simulink model "PID_RS"  (R2019a)
settings: Solver=VariableStepAuto  StartTime=0.0  StopTime=10.0  RelTol=1e-3
values from neighbouring files (symbols this model uses):
  f = 7E-5    (= 7e-05)    [BallOnBeam.m]
  J = 4.6E-5    (= 4.6e-05)    [BallOnBeam.m]
  k = 0.026    [BallOnBeam.m]
  k1 = 7    [BallOnBeam.m]
  k2 = 28.65    [BallOnBeam.m]
  k3 = 0.0159    [BallOnBeam.m]
  kb = 6.1    [BallOnBeam.m]
  ki = 1.6    [BallOnBeam.m]
  kp = nm*J*wndes^2/(k2*k*ki)    (= 27.0462934428)    [BallOnBeam.m]
  kpi = rm*tii*ki/taudesi    (= 1.6)    [BallOnBeam.m]
  kv = (2*xides*J*wndes - f)/(kp*ki*k*k3)    (= 0.093347474441)    [BallOnBeam.m]
  lm = 0.001    [BallOnBeam.m]
  nm = 960    [BallOnBeam.m]
  r0 = x(3)    [BallOnBeam.m]
  r1 = x(4)    [BallOnBeam.m]
  r2 = x(5)    [BallOnBeam.m]
  rm = 0.33    [BallOnBeam.m]
  s1 = x(2)    [BallOnBeam.m]
  Te = 0.2    [BallOnBeam.m]
  tii = 0.5*lm/rm    (= 0.00151515151515)    [BallOnBeam.m]
settings Model: Creator=DELL  LastModifiedBy=DELL

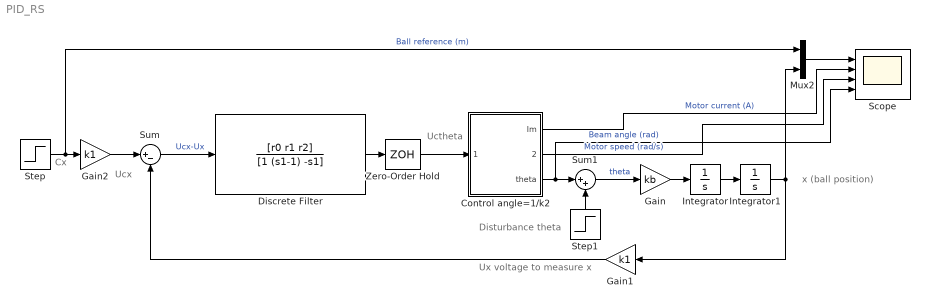
== system PID_RS ==
  note: x (ball position)
  note: Cx
  note: Ucx
  note: Uctheta
  note: Disturbance theta
  note: Ux voltage to measure x
  "Control angle=1/k2 " : Subsystem
  Discrete Filter : DiscreteFilter  Numerator=[r0 r1 r2]  Denominator=[1 (s1-1) -s1]  SampleTime=Te
  Gain : Gain  Gain=kb
  Gain1 : Gain  Gain=k1  SaturateOnIntegerOverflow=on  OutDataTypeStr=Inherit: Same as input  ParamDataTypeStr=Inherit: Same as input
  Gain2 : Gain  Gain=k1  SaturateOnIntegerOverflow=on  OutDataTypeStr=Inherit: Same as input  ParamDataTypeStr=Inherit: Same as input
  Integrator : Integrator
  Integrator1 : Integrator
  Mux2 : Mux  Inputs=2
  Scope : Scope  NumInputPorts=4
  Step : Step  After=0.1  SampleTime=0
  Step1 : Step  Time=10  After=1*pi/180  SampleTime=0
  Sum : Sum  Inputs=|+-  SaturateOnIntegerOverflow=on  InputSameDT=on  OutDataTypeStr=Inherit: Same as first input
  Sum1 : Sum  Inputs=|++  SaturateOnIntegerOverflow=on  InputSameDT=on  OutDataTypeStr=Inherit: Same as first input
  Zero-Order Hold : ZeroOrderHold  SampleTime=-1
  wires:
  "Control angle=1/k2 "/3(theta) -> Scope/4, Sum1/1  "Beam angle (rad)"
  Gain2/1 -> Sum/1
  Step/1 -> Mux2/1, Gain2/1  "Ball reference (m)"
  Step1/1 -> Sum1/2
  Mux2/1 -> Scope/1
  "Control angle=1/k2 "/2(omega) -> Scope/3  "Motor speed (rad/s)"
  "Control angle=1/k2 "/1(Im) -> Scope/2  "Motor current (A)"
  Gain1/1 -> Sum/2
  Discrete Filter/1 -> Zero-Order Hold/1
  Zero-Order Hold/1 -> "Control angle=1/k2 "/1(Uctheta)
  Sum/1 -> Discrete Filter/1  "Ucx-Ux"
  Sum1/1 -> Gain/1  "theta"
  Gain/1 -> Integrator/1
  Integrator1/1 -> Gain1/1, Mux2/2
  Integrator/1 -> Integrator1/1

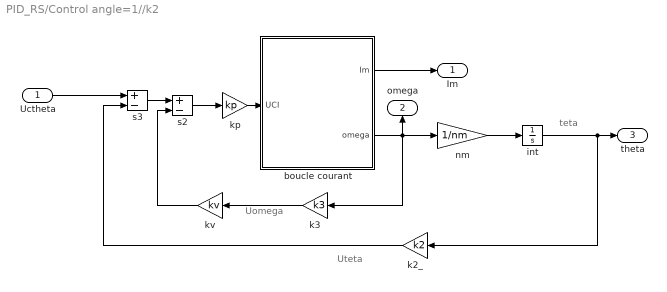
== system PID_RS/Control angle=1//k2  ==
  note: Uomega
  note: teta
  note: Uteta
  Uctheta : Inport
  boucle courant : Subsystem
  int : Integrator
  k2_ : Gain  Gain=k2  SaturateOnIntegerOverflow=on  OutDataTypeStr=Inherit: Same as input  ParamDataTypeStr=Inherit: Same as input
  k3 : Gain  Gain=k3  SaturateOnIntegerOverflow=on  OutDataTypeStr=Inherit: Same as input  ParamDataTypeStr=Inherit: Same as input
  kp : Gain  Gain=kp  SaturateOnIntegerOverflow=on  OutDataTypeStr=Inherit: Same as input  ParamDataTypeStr=Inherit: Same as input
  kv : Gain  Gain=kv  SaturateOnIntegerOverflow=on  OutDataTypeStr=Inherit: Same as input  ParamDataTypeStr=Inherit: Same as input
  nm : Gain  Gain=1/nm  SaturateOnIntegerOverflow=on  OutDataTypeStr=Inherit: Same as input  ParamDataTypeStr=Inherit: Same as input
  s2 : Sum  Inputs=+-  SaturateOnIntegerOverflow=on  InputSameDT=on  OutDataTypeStr=Inherit: Same as first input
  s3 : Sum  Inputs=+-  SaturateOnIntegerOverflow=on  InputSameDT=on  OutDataTypeStr=Inherit: Same as first input
  Im : Outport
  omega : Outport  Port=2
  theta : Outport  Port=3
  wires:
  kp/1 -> boucle courant/1(UCI)
  s2/1 -> kp/1
  s3/1 -> s2/1
  nm/1 -> int/1
  boucle courant/2(omega) -> nm/1, k3/1, omega/1
  k3/1 -> kv/1
  kv/1 -> s2/2
  int/1 -> k2_/1, theta/1
  k2_/1 -> s3/2
  boucle courant/1(Im) -> Im/1
  Uctheta/1 -> s3/1

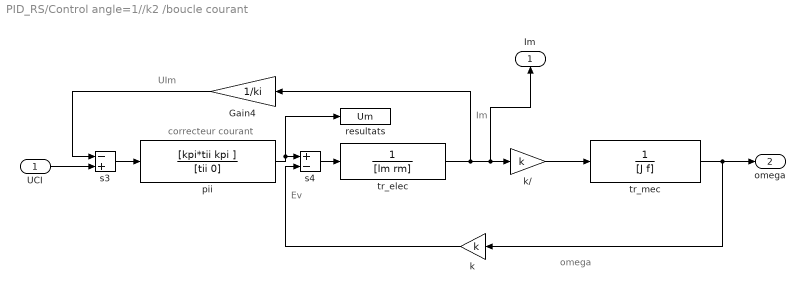
== system PID_RS/Control angle=1//k2 /boucle courant ==
  note: correcteur courant
  note: Im
  note: Ev
  note: UIm
  note: omega
  UCI : Inport
  Gain4 : Gain  Gain=1/ki  SaturateOnIntegerOverflow=on  OutDataTypeStr=Inherit: Same as input  ParamDataTypeStr=Inherit: Same as input
  k : Gain  Gain=k  SaturateOnIntegerOverflow=on  OutDataTypeStr=Inherit: Same as input  ParamDataTypeStr=Inherit: Same as input
  "k/ " : Gain  Gain=k  SaturateOnIntegerOverflow=on  OutDataTypeStr=Inherit: Same as input  ParamDataTypeStr=Inherit: Same as input
  pii : TransferFcn  Numerator=[kpi*tii kpi ]  Denominator=[tii 0]
  resultats : ToWorkspace  VariableName=Um
      settings: MaxDataPoints=20000
  s3 : Sum  Inputs=-+  SaturateOnIntegerOverflow=on  InputSameDT=on  OutDataTypeStr=Inherit: Same as first input
  s4 : Sum  Inputs=+-  SaturateOnIntegerOverflow=on  InputSameDT=on  OutDataTypeStr=Inherit: Same as first input
  tr_elec : TransferFcn  Denominator=[lm rm]
  tr_mec : TransferFcn  Denominator=[J f]
  Im : Outport
  omega : Outport  Port=2
  wires:
  s4/1 -> tr_elec/1
  Gain4/1 -> s3/1
  s3/1 -> pii/1
  k/1 -> s4/2
  "k/ "/1 -> tr_mec/1
  tr_mec/1 -> k/1, omega/1
  UCI/1 -> s3/2
  pii/1 -> s4/1, resultats/1
  tr_elec/1 -> Gain4/1, "k/ "/1, Im/1
